simulink model "lab5_pid"  (R2015b)
settings: Solver=ode45  SolverMode=SingleTasking  StartTime=0.0  StopTime=2  RelTol=1e-3
libraries: truetime x1
settings Model: Creator=peterfj  LastModifiedBy=andfro
settings DataIOCC: SaveFormat=Array
settings OptimizationCC: BlockReduction=off  BooleanDataType=off
settings DebuggingCC: SaveWithParameterizedLinksMsg=none  UnderspecifiedInitializationDetection=Classic  MergeDetectMultiDrivingBlocksExec=none  SignalResolutionControl=TryResolveAllWithWarning
settings HardwareCC: ProdBitPerPointer=32  ProdLargestAtomicFloat=None  ProdIntDivRoundTo=Undefined  ProdEndianess=Unspecified  ProdWordSize=32  ProdHWDeviceType=32-bit Generic  TargetUnknown=on
settings GRTTargetCC: GeneratePreprocessorConditionals=Disable all
settings ConfigComp: CovModelRefEnable=Off  CovSFcnEnable=off

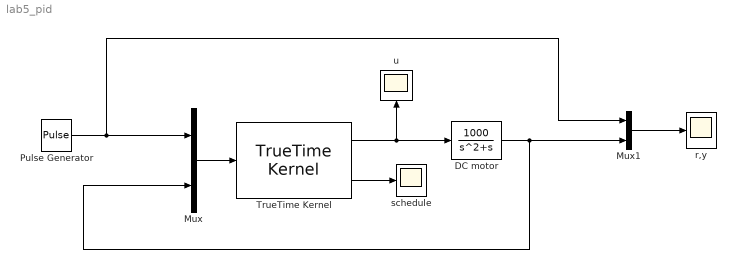
== system lab5_pid ==
  "DC motor " : TransferFcn  Numerator=[1000]  Denominator=[1 1 0]
  Mux : Mux  Inputs=2
  Mux1 : Mux  Inputs=2
  Pulse Generator : DiscretePulseGenerator  PulseType=Time based  Amplitude=2  Period=1  PulseWidth=50  PhaseDelay=0.1  SampleTime=0.005
  TrueTime Kernel : truetime/TrueTime Kernel  sfun=node_init_pid_4  args=1  ninputsoutputs=[2 1]  ntriggers=0  trigtype=falling  nwnodenbr=[]  clockoffsetdrift=[0 0]  schedoutput=on  battery=off  poweroutput=off
  r,y : Scope
  schedule : Scope
  u : Scope
  wires:
  Mux/1 -> TrueTime Kernel/1
  TrueTime Kernel/2 -> schedule/1
  Pulse Generator/1 -> Mux1/1, Mux/1
  "DC motor "/1 -> Mux1/2, Mux/2
  TrueTime Kernel/1 -> "DC motor "/1, u/1
  Mux1/1 -> r,y/1
